simulink model "Simulink_Model"  (R2017a)
settings: Solver=VariableStepAuto  StartTime=0.0  StopTime=50.0  RelTol=1e-3
undefined symbols (not defined in the file): FPI
libraries: fuzblock x1
settings Model: Creator=PRAMADI  LastModifiedBy=PRAMADI

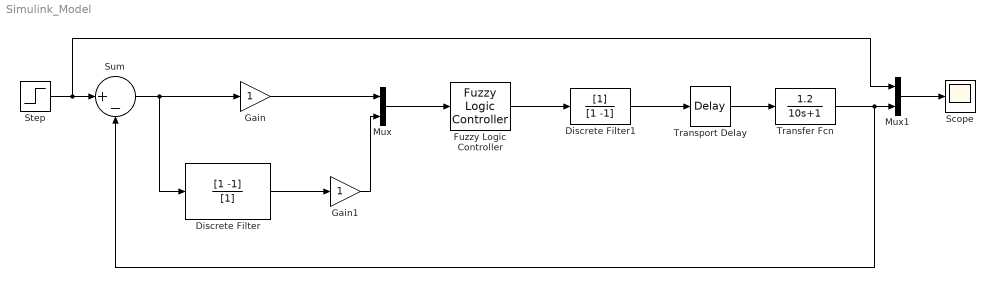
== system Simulink_Model ==
  Discrete Filter : DiscreteFilter  Numerator=[1 -1]  Denominator=[1]  InputProcessing=Columns as channels (frame based)  FilterStructure=Direct form II transposed  a0EqualsOne=on
  Discrete Filter1 : DiscreteFilter  Denominator=[1 -1]
  Fuzzy Logic Controller : fuzblock/Fuzzy Logic  Controller  fis=[FPI]
  Gain : Gain
  Gain1 : Gain
  Mux : Mux  Inputs=2
  Mux1 : Mux  Inputs=2
  Scope : Scope
  Step : Step  SampleTime=0
  Sum : Sum  Inputs=|+-
  Transfer Fcn : TransferFcn  Numerator=[1.2]  Denominator=[10 1]
  Transport Delay : TransportDelay
  wires:
  Sum/1 -> Discrete Filter/1, Gain/1
  Discrete Filter/1 -> Gain1/1
  Gain/1 -> Mux/1
  Gain1/1 -> Mux/2
  Mux/1 -> Fuzzy Logic Controller/1
  Fuzzy Logic Controller/1 -> Discrete Filter1/1
  Discrete Filter1/1 -> Transport Delay/1
  Transport Delay/1 -> Transfer Fcn/1
  Mux1/1 -> Scope/1
  Step/1 -> Mux1/1, Sum/1
  Transfer Fcn/1 -> Sum/2, Mux1/2
